simulink model "rlwatertank_simulation_model6_real"  (R2020b)
settings: Solver=ode45  StartTime=0.0  StopTime=inf  RelTol=1e-3  EnableMultiTasking=on
undefined symbols (not defined in the file or in its folder): DiscIntNeverNeededParam
libraries: simulink x4, opclib x3, rllib x1, sldrtlib x1
settings Model: Creator=The MathWorks, Inc.  LastModifiedBy=Asus
settings DataIOCC: LimitDataPoints=on  SaveFormat=Array  ReturnWorkspaceOutputs=off  SignalLoggingName=logsOut
settings OptimizationCC: ExpressionDepthLimit=2147483647  InitFltsAndDblsToZero=on  LifeSpan=inf
settings DebuggingCC: SignalRangeChecking=error  SaveWithParameterizedLinksMsg=none  UnderspecifiedInitializationDetection=Classic  MergeDetectMultiDrivingBlocksExec=none  SignalResolutionControl=TryResolveAllWithWarning  MultiTaskDSMMsg=warning  FcnCallInpInsideContextMsg=warning  AllowSymbolicDim=off  StateNameClashWarn=warning  SFUnexpectedBacktrackingDiag=warning  SFNoUnconditionalDefaultTransitionDiag=warning  SFExecutionAtInitializationDiag=none  ArithmeticOperatorsInVariantConditions=warning
settings HardwareCC: ProdBitPerPointer=32  ProdBitPerSizeT=32  ProdBitPerPtrDiffT=32  ProdLargestAtomicFloat=None  ProdIntDivRoundTo=Undefined  ProdEndianess=Unspecified  ProdWordSize=32  ProdHWDeviceType=Specified
settings ModelReferenceCC: PropagateSignalLabelsOutOfModel=off
settings SFSimCC: SimUseLocalCustomCode=off  CustomCodeUndefinedFunction=UseInterfaceOnly
settings RTWCC: RTWUseLocalCustomCode=off
settings CodeAppCC: StateflowObjectComments=on
settings GRTTargetCC: TargetFcnLib=ansi_tfl_tmw.mat  TargetLangStandard=C89/C90 (ANSI)  CombineOutputUpdateFcns=off  GRTInterface=on
settings ConfigComp: CovMetricSettings=dw  CovSaveCumulativeToWorkspaceVar=on  CovSaveSingleToWorkspaceVar=on  CovExternalEMLEnable=off

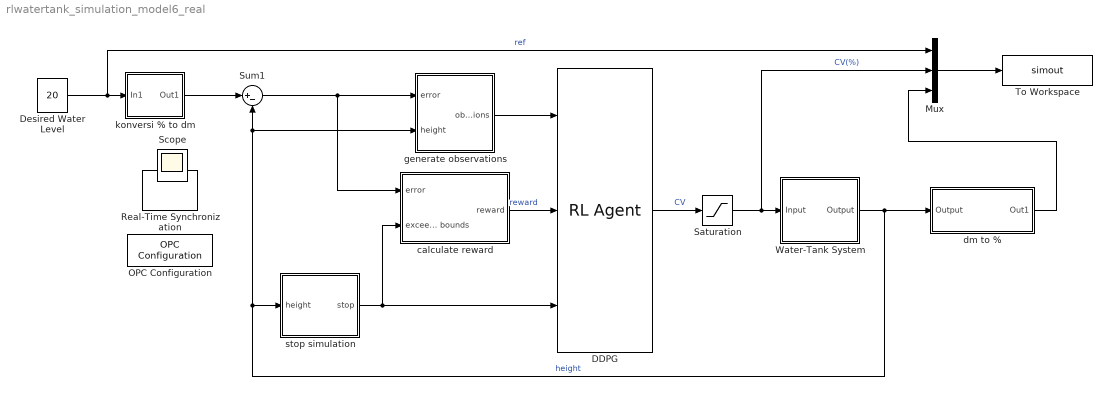
== system rlwatertank_simulation_model6_real ==
  DDPG : rllib/RL Agent  Agent=agent  ProvideReward=on  ProvideIsDone=on  ProvideCumRwd=off  TreatAsDirectFeedthrough=on  CollectLoggedSignals=on  CollectModelStates=on
      settings: SourceProductName=Reinforcement Learning
  Desired Water Level : Constant  Value=20
  Mux : Mux  Inputs=3
  OPC Configuration : opclib/OPC Configuration  opcServers=localhost/KEPware.KEPServerEx.V4/10  errMissingItems=Error  errReadWrite=Warn  errShutdown=Error  errRTViolation=Warn  rtEnable=on  speedup=1  showLatency=off  beingUsed=on
      settings: SourceProductBaseCode=OT
  Real-Time Synchronization : sldrtlib/Real-Time Synchronization  SampleTime=0.1  MaxMissedTicks=10  ShowMissedTicks=off  YieldWhenWaiting=off
  Saturation : Saturate  UpperLimit=100  LowerLimit=0  ZeroCross=off  OutMin=0  OutMax=100
  Sum1 : Sum  Inputs=|+-  SaturateOnIntegerOverflow=on
  To Workspace : ToWorkspace  VariableName=simout  SaveFormat=Timeseries  SampleTime=-1
  Water-Tank System : Subsystem
  calculate reward : Subsystem
  dm to % : Subsystem
  generate observations : Subsystem
  konversi % to dm : Subsystem
  stop simulation : Subsystem
  Scope : Scope
  wires:
  Sum1/1 -> calculate reward/1(error), generate observations/1(error)
  Water-Tank System/1(Output) -> stop simulation/1(height), generate observations/2(height), Sum1/2, dm to %/1(Output)  "height"
  stop simulation/1(stop) -> DDPG/3, calculate reward/2(exceeds bounds)
  calculate reward/1(reward) -> DDPG/2  "reward"
  generate observations/1(observations) -> DDPG/1
  Saturation/1 -> Mux/2, Water-Tank System/1(Input)  "CV(%)"
  Mux/1 -> To Workspace/1
  DDPG/1 -> Saturation/1  "CV"
  Desired Water Level/1 -> Mux/1, konversi % to dm/1(In1)  "ref"
  konversi % to dm/1(Out1) -> Sum1/1
  dm to %/1(Out1) -> Mux/3

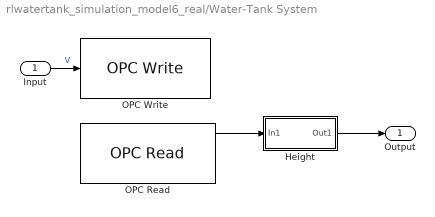
== system rlwatertank_simulation_model6_real/Water-Tank System ==
  Input : Inport
  Height : Subsystem
  OPC Read : opclib/OPC Read  serverHost=localhost  serverID=KEPware.KEPServerEx.V4  itemIDs=Fultek.CPU101F.LVL  readMode=Synchronous (cache)  dataType=double  updateRate=0.1  showQual=on  showTS=on  tsMode=Seconds since start
      settings: SourceProductBaseCode=OT
  OPC Write : opclib/OPC Write  serverHost=localhost  serverID=KEPware.KEPServerEx.V4  itemIDs=Fultek.CPU101F.ControlValve  writeMode=Synchronous  updateRate=0
      settings: SourceProductBaseCode=OT
  Output : Outport  VectorParamsAs1DForOutWhenUnconnected=off
  wires:
  Input/1 -> OPC Write/1  "V"
  Height/1(Out1) -> Output/1
  OPC Read/1 -> Height/1(In1)

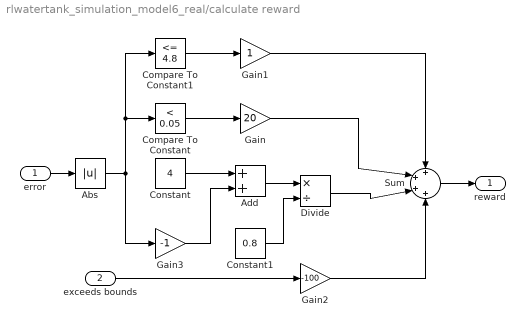
== system rlwatertank_simulation_model6_real/calculate reward ==
  error : Inport
  exceeds bounds : Inport  Port=2
  Abs : Abs  ZeroCross=off
  Add : Sum
  Compare To Constant : simulink/Logic and Bit Operations/Compare To Constant  relop=<  const=0.05  OutDataTypeStr=boolean  ZeroCross=off
  Compare To Constant1 : simulink/Logic and Bit Operations/Compare To Constant  relop=<=  const=4.8  OutDataTypeStr=boolean  ZeroCross=off
  Constant : Constant  Value=4
  Constant1 : Constant  Value=0.8
  Divide : Product  Inputs=*/
  Gain : Gain  Gain=20
  Gain1 : Gain
  Gain2 : Gain  Gain=-100
  Gain3 : Gain  Gain=-1
  Sum : Sum  Inputs=++++  OutDataTypeStr=double
  reward : Outport  VectorParamsAs1DForOutWhenUnconnected=off
  wires:
  Gain2/1 -> Sum/4
  Gain/1 -> Sum/2
  Compare To Constant/1 -> Gain/1
  Sum/1 -> reward/1
  exceeds bounds/1 -> Gain2/1
  error/1 -> Abs/1
  Abs/1 -> Gain3/1, Compare To Constant1/1, Compare To Constant/1
  Compare To Constant1/1 -> Gain1/1
  Gain1/1 -> Sum/1
  Constant/1 -> Add/1
  Gain3/1 -> Add/2
  Add/1 -> Divide/1
  Constant1/1 -> Divide/2
  Divide/1 -> Sum/3

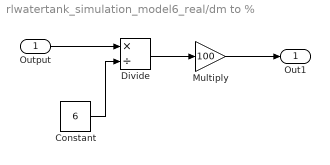
== system rlwatertank_simulation_model6_real/dm to % ==
  Output : Inport
  Constant : Constant  Value=6
  Divide : Product  Inputs=*/
  Multiply : Gain  Gain=100
  Out1 : Outport
  wires:
  Output/1 -> Divide/1
  Constant/1 -> Divide/2
  Divide/1 -> Multiply/1
  Multiply/1 -> Out1/1

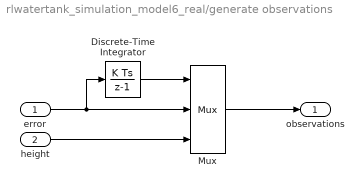
== system rlwatertank_simulation_model6_real/generate observations ==
  error : Inport
  height : Inport  Port=2
  Discrete-Time Integrator : DiscreteIntegrator  ICPrevOutput=DiscIntNeverNeededParam  ICPrevScaledInput=DiscIntNeverNeededParam
  Mux : Mux  Inputs=3
  observations : Outport  VectorParamsAs1DForOutWhenUnconnected=off
  wires:
  height/1 -> Mux/3
  Discrete-Time Integrator/1 -> Mux/1
  error/1 -> Discrete-Time Integrator/1, Mux/2
  Mux/1 -> observations/1

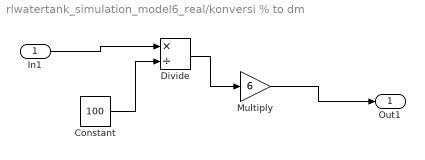
== system rlwatertank_simulation_model6_real/konversi % to dm ==
  In1 : Inport
  Constant : Constant  Value=100
  Divide : Product  Inputs=*/
  Multiply : Gain  Gain=6
  Out1 : Outport
  wires:
  In1/1 -> Divide/1
  Constant/1 -> Divide/2
  Divide/1 -> Multiply/1
  Multiply/1 -> Out1/1

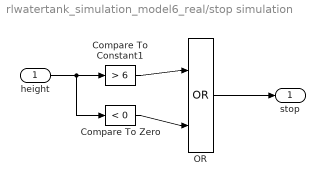
== system rlwatertank_simulation_model6_real/stop simulation ==
  height : Inport
  Compare To Constant1 : simulink/Logic and Bit Operations/Compare To Constant  relop=>  const=6  OutDataTypeStr=boolean  ZeroCross=off
  Compare To Zero : simulink/Logic and Bit Operations/Compare To Zero  relop=<  OutDataTypeStr=boolean  ZeroCross=off
  OR : Logic  Operator=OR  IconShape=distinctive  AllPortsSameDT=off  OutDataTypeStr=boolean
  stop : Outport  VectorParamsAs1DForOutWhenUnconnected=off
  wires:
  height/1 -> Compare To Zero/1, Compare To Constant1/1
  Compare To Zero/1 -> OR/2
  Compare To Constant1/1 -> OR/1
  OR/1 -> stop/1

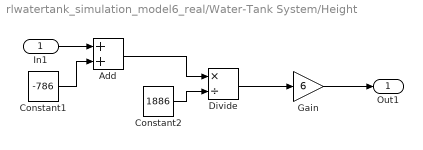
== system rlwatertank_simulation_model6_real/Water-Tank System/Height ==
  In1 : Inport
  Add : Sum
  Constant1 : Constant  Value=-786
  Constant2 : Constant  Value=1886
  Divide : Product  Inputs=*/
  Gain : Gain  Gain=6
  Out1 : Outport
  wires:
  Add/1 -> Divide/1
  Divide/1 -> Gain/1
  Constant1/1 -> Add/2
  Constant2/1 -> Divide/2
  In1/1 -> Add/1
  Gain/1 -> Out1/1
